simulink model "E_Simulacao_Simulink"  (R2019a)
settings: Solver=VariableStepAuto  StartTime=0.0  StopTime=346  RelTol=1e-3
values from neighbouring files (symbols this model uses):
  A = [yv (yp+aa0) (yr - 1) (g*cos(tt0)/u0); l_lv l_lp l_lr 0; n_lv n_lp n_lr 0; 0 1 tan(tt0) 0]    [A_Anel_Aberto.m]    (also in B_SISO.m; C_D_LQR_e_Sensores.m = [yv (yp+aa0) (yr - 1) (g*cos(tt0)/u0) 0; l_lv l_lp l_lr 0 0;)
  B = [Yda Ydr ; Lda Ldr ; Nda Ndr ; 0 0]    [A_Anel_Aberto.m]    (also in B_SISO.m; C_D_LQR_e_Sensores.m = [Yda Ydr ; Lda Ldr ; Nda Ndr ; 0 0; 0 0])
  C = [1 0 0 0 ; 0 1 0 0 ; 0 0 1 0 ; 0 0 0 1]    [A_Anel_Aberto.m]    (also in B_SISO.m; C_D_LQR_e_Sensores.m = [1 0 0 0 0; 0 1 0 0 0; 0 0 1 0 0; 0 0 0 1 0; 0 0 0 0 1])
  D = [0 0; 0 0; 0 0; 0 0]    [A_Anel_Aberto.m]    (also in B_SISO.m; C_D_LQR_e_Sensores.m = [0 0; 0 0; 0 0; 0 0; 0 0])
  deg = pi/180    (= 0.0174532777778)    [A_Anel_Aberto.m]    (also in B_SISO.m; C_D_LQR_e_Sensores.m)
  K = lqr(A,B,Q,R)    [C_D_LQR_e_Sensores.m]
  u0 = 84.99    [A_Anel_Aberto.m]    (also in B_SISO.m; C_D_LQR_e_Sensores.m)
libraries: simulink x6
settings Model: Creator=Antonio Oliveira  LastModifiedBy=Antonio Oliveira

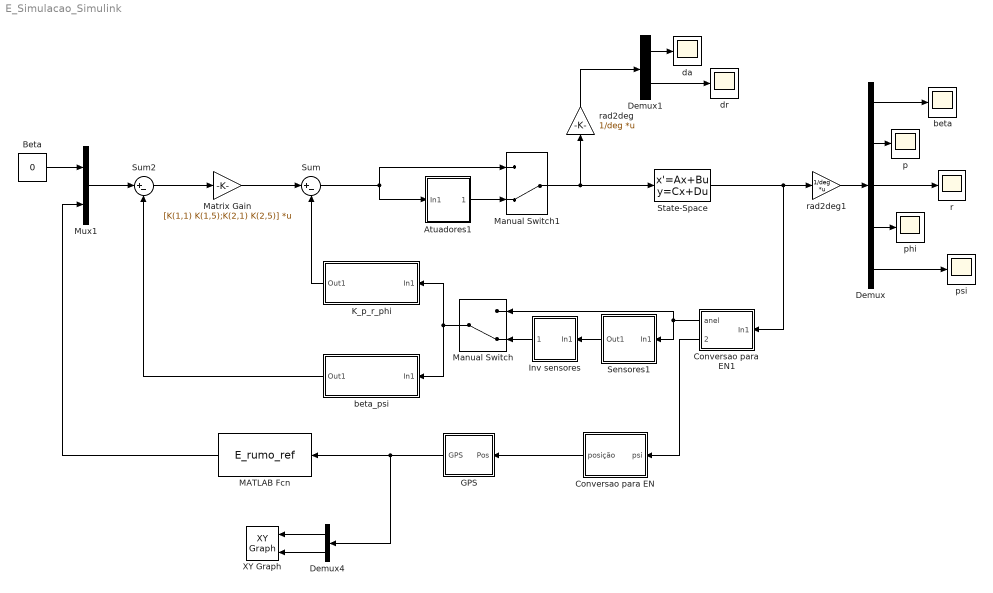
== system E_Simulacao_Simulink ==
  Atuadores1 : Subsystem
  Beta : Constant  Value=0
  Conversao para EN : Subsystem
  Conversao para EN1 : Subsystem
  Demux : Demux  Outputs=5
  Demux1 : Demux  Outputs=2
  Demux4 : Demux  Outputs=2
  GPS : Subsystem
  Inv sensores : Subsystem
  K_p_r_phi : Subsystem
  MATLAB Fcn : MATLABFcn  MATLABFcn=E_rumo_ref  OutputDimensions=1  OutputSignalType=real
  Manual Switch : ManualSwitch  CurrentSetting=0
  Manual Switch1 : ManualSwitch  CurrentSetting=0
  Matrix Gain : Gain  Gain=[K(1,1) K(1,5);K(2,1) K(2,5)]  Multiplication=Matrix(K*u)  SaturateOnIntegerOverflow=on  OutDataTypeStr=Inherit: Same as input  ParamDataTypeStr=Inherit: Same as input
  Mux1 : Mux  Inputs=2
  Sensores1 : Subsystem
  State-Space : StateSpace  A=A  B=B  C=C  D=D  InitialCondition=[0, 0, 0, 0, 45*deg]
  Sum : Sum  Inputs=|+-  SaturateOnIntegerOverflow=on  InputSameDT=on  OutDataTypeStr=Inherit: Same as first input
  Sum2 : Sum  Inputs=|+-  SaturateOnIntegerOverflow=on  InputSameDT=on  OutDataTypeStr=Inherit: Same as first input
  XY Graph : simulink/Sinks/XY Graph  xmin=-4e2  xmax=7e3  ymin=-3e3  ymax=8e3  st=-1
  beta : Scope
  beta_psi : Subsystem
  da : Scope
  dr : Scope
  p : Scope
  phi : Scope
  psi : Scope
  r : Scope
  rad2deg : Gain  Gain=1/deg  Multiplication=Matrix(K*u)  SaturateOnIntegerOverflow=on  OutDataTypeStr=Inherit: Same as input  ParamDataTypeStr=Inherit: Same as input
  rad2deg1 : Gain  Gain=1/deg  Multiplication=Matrix(K*u)  SaturateOnIntegerOverflow=on  OutDataTypeStr=Inherit: Same as input  ParamDataTypeStr=Inherit: Same as input
  wires:
  Demux/5 -> psi/1
  Matrix Gain/1 -> Sum/1
  Demux1/1 -> da/1
  Demux/2 -> p/1
  Manual Switch1/1 -> State-Space/1, rad2deg/1
  rad2deg/1 -> Demux1/1
  Demux1/2 -> dr/1
  Sum/1 -> Atuadores1/1(In1), Manual Switch1/1
  rad2deg1/1 -> Demux/1
  Manual Switch/1 -> beta_psi/1(In1), K_p_r_phi/1(In1)
  State-Space/1 -> Conversao para EN1/1(In1), rad2deg1/1
  K_p_r_phi/1(Out1) -> Sum/2
  beta_psi/1(Out1) -> Sum2/2
  Demux/4 -> phi/1
  Demux/3 -> r/1
  Inv sensores/1(Out1) -> Manual Switch/2
  Demux/1 -> beta/1
  Mux1/1 -> Sum2/1
  Beta/1 -> Mux1/1
  Conversao para EN1/1(anel) -> Sensores1/1(In1), Manual Switch/1
  Conversao para EN1/2(Posição) -> Conversao para EN/1(psi)
  Conversao para EN/1(posição) -> GPS/1(Pos)
  Sensores1/1(Out1) -> Inv sensores/1(In1)
  Atuadores1/1(Out1) -> Manual Switch1/2
  Demux4/2 -> XY Graph/2
  GPS/1(GPS) -> Demux4/1, MATLAB Fcn/1
  Demux4/1 -> XY Graph/1
  Sum2/1 -> Matrix Gain/1
  MATLAB Fcn/1 -> Mux1/2

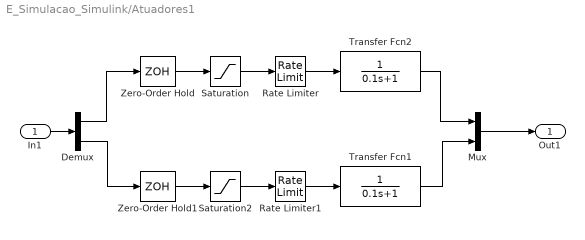
== system E_Simulacao_Simulink/Atuadores1 ==
  In1 : Inport
  Demux : Demux  Outputs=2
  Mux : Mux  Inputs=2
  Rate Limiter : RateLimiter  SampleTimeMode=inherited
  Rate Limiter1 : RateLimiter  SampleTimeMode=inherited
  Saturation : Saturate  UpperLimit=17*deg  LowerLimit=-17*deg
  Saturation2 : Saturate  UpperLimit=23*deg  LowerLimit=-23*deg
  Transfer Fcn1 : TransferFcn  Denominator=[0.1 1]
  Transfer Fcn2 : TransferFcn  Denominator=[0.1 1]
  Zero-Order Hold : ZeroOrderHold  SampleTime=0.025
  Zero-Order Hold1 : ZeroOrderHold  SampleTime=0.025
  Out1 : Outport
  wires:
  Demux/1 -> Zero-Order Hold/1
  Demux/2 -> Zero-Order Hold1/1
  In1/1 -> Demux/1
  Saturation2/1 -> Rate Limiter1/1
  Mux/1 -> Out1/1
  Zero-Order Hold1/1 -> Saturation2/1
  Zero-Order Hold/1 -> Saturation/1
  Rate Limiter/1 -> Transfer Fcn2/1
  Saturation/1 -> Rate Limiter/1
  Transfer Fcn2/1 -> Mux/1
  Rate Limiter1/1 -> Transfer Fcn1/1
  Transfer Fcn1/1 -> Mux/2

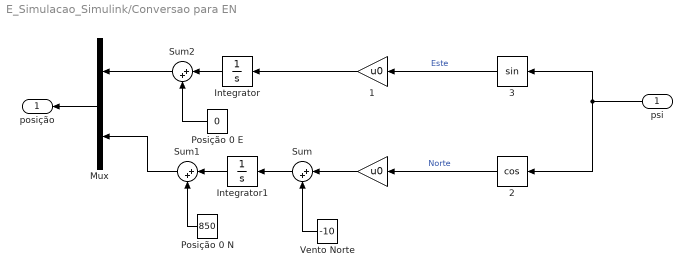
== system E_Simulacao_Simulink/Conversao para EN ==
  psi : Inport
  " " : Gain  Gain=u0
  " 1" : Gain  Gain=u0
  " 2" : Trigonometry  Operator=cos
  " 3" : Trigonometry
  Integrator : Integrator
  Integrator1 : Integrator
  Mux : Mux  Inputs=2
  Posição 0 E : Constant  Value=0
  Posição 0 N : Constant  Value=850
  Sum : Sum  Inputs=|++
  Sum1 : Sum  Inputs=|++
  Sum2 : Sum  Inputs=|++
  Vento Norte : Constant  Value=-10
  posição : Outport
  wires:
  psi/1 -> " 3"/1, " 2"/1
  " 3"/1 -> " 1"/1  "Este"
  " 2"/1 -> " "/1  "Norte"
  " 1"/1 -> Integrator/1
  " "/1 -> Sum/1
  Vento Norte/1 -> Sum/2
  Sum/1 -> Integrator1/1
  Mux/1 -> posição/1
  Integrator/1 -> Sum2/1
  Integrator1/1 -> Sum1/1
  Sum2/1 -> Mux/1
  Sum1/1 -> Mux/2
  Posição 0 E/1 -> Sum2/2
  Posição 0 N/1 -> Sum1/2

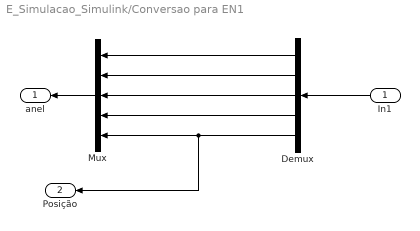
== system E_Simulacao_Simulink/Conversao para EN1 ==
  In1 : Inport
  Demux : Demux  Outputs=5
  Mux : Mux  Inputs=5
  anel : Outport
  Posição : Outport  Port=2
  wires:
  In1/1 -> Demux/1
  Demux/1 -> Mux/1
  Demux/2 -> Mux/2
  Demux/4 -> Mux/4
  Demux/5 -> Mux/5, Posição/1
  Demux/3 -> Mux/3
  Mux/1 -> anel/1

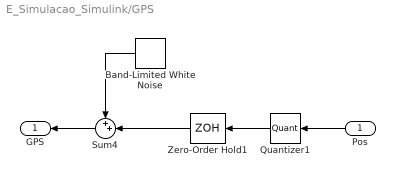
== system E_Simulacao_Simulink/GPS ==
  Pos : Inport
  "Band-Limited White Noise " : simulink/Sources/Band-Limited White Noise  Cov=[4^2]  Ts=1  seed=[23341]
  Quantizer1 : Quantizer
  Sum4 : Sum  Inputs=++|
  Zero-Order Hold1 : ZeroOrderHold
  GPS : Outport
  wires:
  Zero-Order Hold1/1 -> Sum4/2
  "Band-Limited White Noise "/1 -> Sum4/1
  Quantizer1/1 -> Zero-Order Hold1/1
  Pos/1 -> Quantizer1/1
  Sum4/1 -> GPS/1

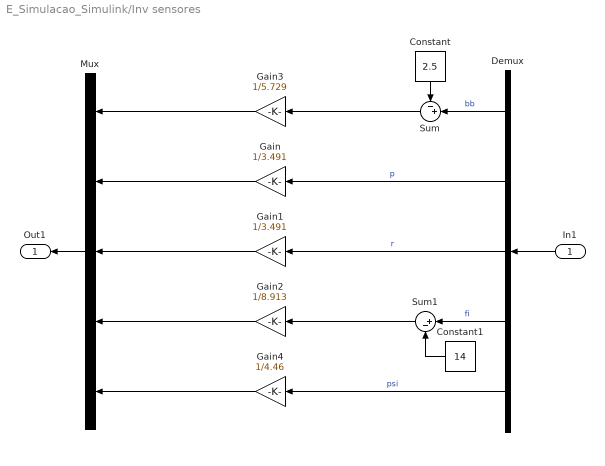
== system E_Simulacao_Simulink/Inv sensores ==
  In1 : Inport
  Constant : Constant  Value=2.5
  Constant1 : Constant  Value=14
  Demux : Demux  Outputs=5
  Gain : Gain  Gain=1/3.491
  Gain1 : Gain  Gain=1/3.491
  Gain2 : Gain  Gain=1/8.913
  Gain3 : Gain  Gain=1/5.729
  Gain4 : Gain  Gain=1/4.46
  Mux : Mux  Inputs=5
  Sum : Sum  Inputs=-+|
  Sum1 : Sum  Inputs=|+-
  Out1 : Outport
  wires:
  Mux/1 -> Out1/1
  In1/1 -> Demux/1
  Demux/1 -> Sum/2  "bb"
  Demux/2 -> Gain/1  "p"
  Demux/3 -> Gain1/1  "r"
  Demux/4 -> Sum1/1  "fi"
  Constant/1 -> Sum/1
  Constant1/1 -> Sum1/2
  Sum1/1 -> Gain2/1
  Sum/1 -> Gain3/1
  Gain2/1 -> Mux/4
  Gain1/1 -> Mux/3
  Gain/1 -> Mux/2
  Gain3/1 -> Mux/1
  Demux/5 -> Gain4/1  "psi"
  Gain4/1 -> Mux/5

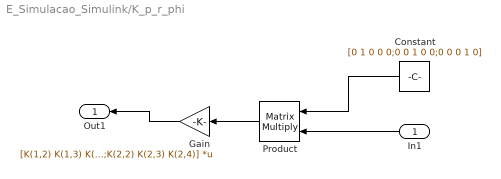
== system E_Simulacao_Simulink/K_p_r_phi ==
  In1 : Inport
  Constant : Constant  Value=[0 1 0 0 0;0 0 1 0 0;0 0 0 1 0]  VectorParams1D=off
  Gain : Gain  Gain=[K(1,2) K(1,3) K(1,4);K(2,2) K(2,3) K(2,4)]  Multiplication=Matrix(K*u)
  Product : Product  Multiplication=Matrix(*)  RndMeth=Zero
  Out1 : Outport
  wires:
  In1/1 -> Product/2
  Constant/1 -> Product/1
  Product/1 -> Gain/1
  Gain/1 -> Out1/1

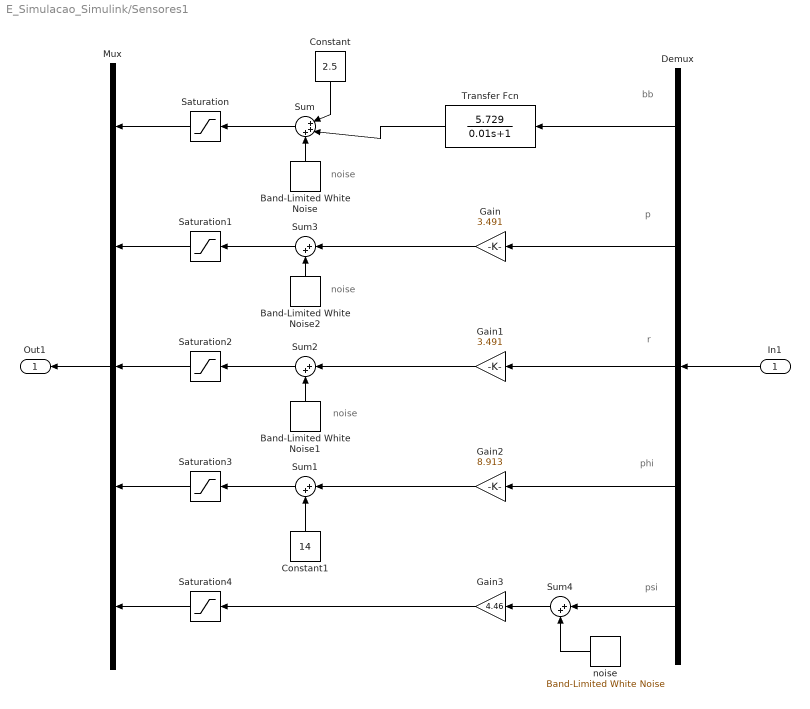
== system E_Simulacao_Simulink/Sensores1 ==
  note: psi
  note: noise
  note: phi
  note: p
  note: r
  note: bb
  note: noise
  note: noise
  In1 : Inport
  Band-Limited White Noise : simulink/Sources/Band-Limited White Noise  Cov=[0.000000625]  Ts=0.025  seed=[23331]
  Band-Limited White Noise1 : simulink/Sources/Band-Limited White Noise  Cov=[0.0000001]  Ts=0.025  seed=[23541]
  Band-Limited White Noise2 : simulink/Sources/Band-Limited White Noise  Cov=[0.0000001]  Ts=0.025  seed=[23344]
  Constant : Constant  Value=2.5
  Constant1 : Constant  Value=14
  Demux : Demux  Outputs=5
  Gain : Gain  Gain=3.491
  Gain1 : Gain  Gain=3.491
  Gain2 : Gain  Gain=8.913
  Gain3 : Gain  Gain=4.46
  Mux : Mux  Inputs=5
  Saturation : Saturate  UpperLimit=5  LowerLimit=0
  Saturation1 : Saturate  UpperLimit=3  LowerLimit=-3
  Saturation2 : Saturate  UpperLimit=3  LowerLimit=-3
  Saturation3 : Saturate  UpperLimit=28  LowerLimit=0
  Saturation4 : Saturate  UpperLimit=28  LowerLimit=0
  Sum : Sum  Inputs=|+++
  Sum{1..4} (4 alike) : Sum  Inputs=|++
  Transfer Fcn : TransferFcn  Numerator=[5.729]  Denominator=[0.01 1]
  noise : simulink/Sources/Band-Limited White Noise  Cov=[0.0000171]  Ts=0.025  seed=[18341]
  Out1 : Outport
  wires:
  Constant1/1 -> Sum1/2
  Demux/4 -> Gain2/1
  Band-Limited White Noise/1 -> Sum/3
  Band-Limited White Noise2/1 -> Sum3/2
  Gain2/1 -> Sum1/1
  Demux/3 -> Gain1/1
  Demux/2 -> Gain/1
  Demux/1 -> Transfer Fcn/1
  Constant/1 -> Sum/1
  In1/1 -> Demux/1
  Mux/1 -> Out1/1
  Gain3/1 -> Saturation4/1
  Sum4/1 -> Gain3/1
  noise/1 -> Sum4/2
  Saturation4/1 -> Mux/5
  Demux/5 -> Sum4/1
  Transfer Fcn/1 -> Sum/2
  Sum/1 -> Saturation/1
  Saturation/1 -> Mux/1
  Gain/1 -> Sum3/1
  Sum3/1 -> Saturation1/1
  Saturation1/1 -> Mux/2
  Sum2/1 -> Saturation2/1
  Saturation2/1 -> Mux/3
  Gain1/1 -> Sum2/1
  Band-Limited White Noise1/1 -> Sum2/2
  Sum1/1 -> Saturation3/1
  Saturation3/1 -> Mux/4

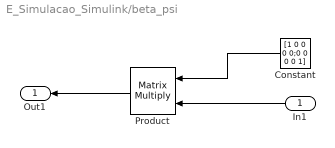
== system E_Simulacao_Simulink/beta_psi ==
  In1 : Inport
  Constant : Constant  Value=[1 0 0 0 0;0 0 0 0 1]  VectorParams1D=off
  Product : Product  Multiplication=Matrix(*)  RndMeth=Zero
  Out1 : Outport
  wires:
  Constant/1 -> Product/1
  Product/1 -> Out1/1
  In1/1 -> Product/2
